simulink model "simple_control_system_controlled_discreet_saturation"  (R2016b)
settings: Solver=VariableStepAuto  StartTime=0.0  StopTime=2  RelTol=1e-3
values from neighbouring files (symbols this model uses):
  Kp1 = 0.1    [simple_control_system_matlab.m]
  Ks = 100    [simulink_parameter.m]
  R2z = c2d(R2,Ts)    [simple_control_system_matlab.m]
  taua = 1e-3    (= 0.001)    [simulink_parameter.m]
  taup = 100e-3    (= 0.1)    [simulink_parameter.m]
  taus = 100e-6    (= 0.0001)    [simulink_parameter.m]
  Ts = 1/fs    (= 0.01)    [simple_control_system_matlab.m]
undefined symbols (not defined in the file or in its folder): U_in, U_sat_max, U_sat_min
settings Model: Creator=lapmint  LastModifiedBy=lapmint

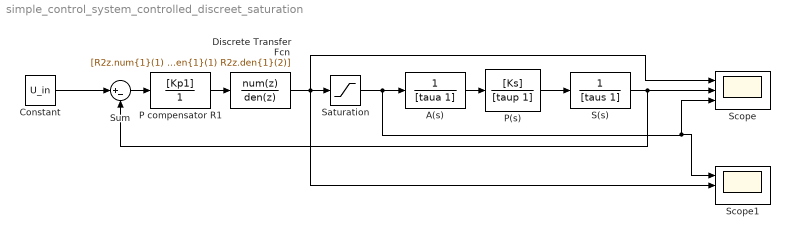
== system simple_control_system_controlled_discreet_saturation ==
  A(s) : TransferFcn  Denominator=[taua 1]
  Constant : Constant  Value=U_in
  Discrete Transfer Fcn : DiscreteTransferFcn  Numerator=[R2z.num{1}(1) R2z.num{1}(2)]  Denominator=[R2z.den{1}(1) R2z.den{1}(2)]  SampleTime=Ts
  P compensator R1 : TransferFcn  Numerator=[Kp1]  Denominator=[0 1]
  P(s) : TransferFcn  Numerator=[Ks]  Denominator=[taup 1]
  S(s) : TransferFcn  Denominator=[taus 1]
  Saturation : Saturate  UpperLimit=U_sat_max  LowerLimit=U_sat_min
  Scope : Scope  NumInputPorts=3
  Scope1 : Scope  NumInputPorts=3
  Sum : Sum  Inputs=|+-
  wires:
  A(s)/1 -> P(s)/1
  P(s)/1 -> S(s)/1
  Constant/1 -> Sum/1
  P compensator R1/1 -> Discrete Transfer Fcn/1
  Discrete Transfer Fcn/1 -> Scope1/2, Scope/1, Saturation/1
  Sum/1 -> P compensator R1/1
  S(s)/1 -> Scope/2, Sum/2
  Saturation/1 -> Scope1/1, Scope/3, A(s)/1
